simulink model "localization"  (R2019b)
settings: Solver=FixedStepAuto  StartTime=0.0  StopTime=310  FixedStep=sample_time  RelTol=1e-3
PreLoadFcn:
  | initLocalization
InitFcn:
  | initLocalization
  | insertArtificialOutages
StopFcn:
  | simout_data_prepared = false;
  | map_data_prepared = false;
  | % prepareSimOutData
undefined symbols (not defined in the file or in its folder): a_bias_gain, a_e_limit, a_e_ma_time, d_bogies, E_w_limit, E_w_ma_time, gnss_lever_arm, gnss_sample_time, gnss_speed_limit, imm_sample_time, p_llh_n_0_rad, psi_0, Q_arc, q_b_n_0, Q_imm, Q_imm_trash, Q_straight, sample_time, sigma_v_acc, sigma_v_gyro, v_min_tgc, v_ned_eb_n_0, w_bias_gain
libraries: libMdl_RecordedData x4, libMdl_quatToEuler x3, simulink x2, libMdl_InsBiasEstimator x2, libMdl_Imm x1, libMdl_KalmanFilter x1, libMdl_invQuat x1, libMdl_GnssDataCorrector x1, libMdl_ImuDataCorrector x1, libMdl_AccIntegrator x1, libMdl_AttitudeComputer x1, libMdl_CarriageMisalignment x1
(part 1 of 2)
settings Model: PauseTimes=14.4  Creator=Hanno  LastModifiedBy=wint_hn
settings SolverCC: AutoInsertRateTranBlk=on
settings DataIOCC: SaveOutput=off  SignalLogging=off  DSMLogging=off  SaveTime=off  ReturnWorkspaceOutputs=off

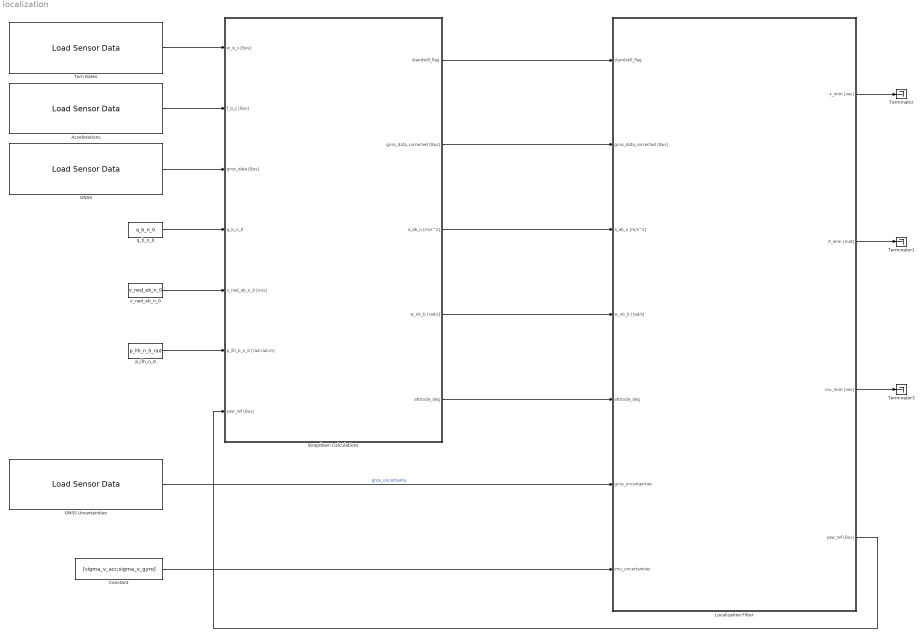
== system localization ==
  Accelerations : libMdl_RecordedData/Load Sensor Data  mv_input_data=acc_data  mv_data_validity=acc_data_validity  mv_input_time=time_imu  mv_sample_time=imu_sample_time
  Constant : Constant  Value=[sigma_v_acc;sigma_v_gyro]
  GNSS : libMdl_RecordedData/Load Sensor Data  mv_input_data=gnss_sim_data  mv_data_validity=gnss_sim_data_validity  mv_input_time=time_gnss  mv_sample_time=gnss_sample_time
  GNSS Uncertainties : libMdl_RecordedData/Load Sensor Data  mv_input_data=gnss_uncertainty_sim_data  mv_data_validity=gnss_sim_data_validity  mv_input_time=time_gnss  mv_sample_time=gnss_sample_time
  Localization Filter : Subsystem
  Strapdown Calculations : Subsystem
  Terminator : Terminator
  Terminator1 : Terminator
  Terminator3 : Terminator
  Turn Rates : libMdl_RecordedData/Load Sensor Data  mv_input_data=gyro_data  mv_data_validity=gyro_data_validity  mv_input_time=time_imu  mv_sample_time=imu_sample_time
  p_llh_n_0 : Constant  Value=p_llh_n_0_rad
  q_b_n_0 : Constant  Value=q_b_n_0
  v_ned_eb_n_0 : Constant  Value=v_ned_eb_n_0
  wires:
  Turn Rates/1 -> Strapdown Calculations/1(w_is_s [Bus])
  Accelerations/1 -> Strapdown Calculations/2(f_is_s [Bus])
  GNSS/1 -> Strapdown Calculations/3(gnss_data [Bus])
  q_b_n_0/1 -> Strapdown Calculations/4(q_b_n_0)
  v_ned_eb_n_0/1 -> Strapdown Calculations/5(v_ned_eb_n_0 [m/s])
  p_llh_n_0/1 -> Strapdown Calculations/6(p_llh_b_n_0 [rad,rad,m])
  Strapdown Calculations/2(gnss_data_corrected [Bus]) -> Localization Filter/2(gnss_data_corrected [Bus])
  GNSS Uncertainties/1 -> Localization Filter/6(gnss_uncertainties)  "gnss_uncertainty"
  Constant/1 -> Localization Filter/7(imu_uncertainties)
  Localization Filter/1(x_imm [vec]) -> Terminator/1
  Localization Filter/2(P_imm [mat]) -> Terminator1/1
  Localization Filter/3(mu_imm [vec]) -> Terminator3/1
  Strapdown Calculations/1(standstill_flag) -> Localization Filter/1(standstill_flag)
  Strapdown Calculations/3(a_eb_n [m/s^2]) -> Localization Filter/3(a_eb_n [m/s^2])
  Strapdown Calculations/4(w_nb_b [rad/s]) -> Localization Filter/4(w_nb_b [rad/s])
  Localization Filter/4(yaw_ref [Bus]) -> Strapdown Calculations/7(yaw_ref [Bus])
  Strapdown Calculations/5(attitude_deg) -> Localization Filter/5(attitude_deg)

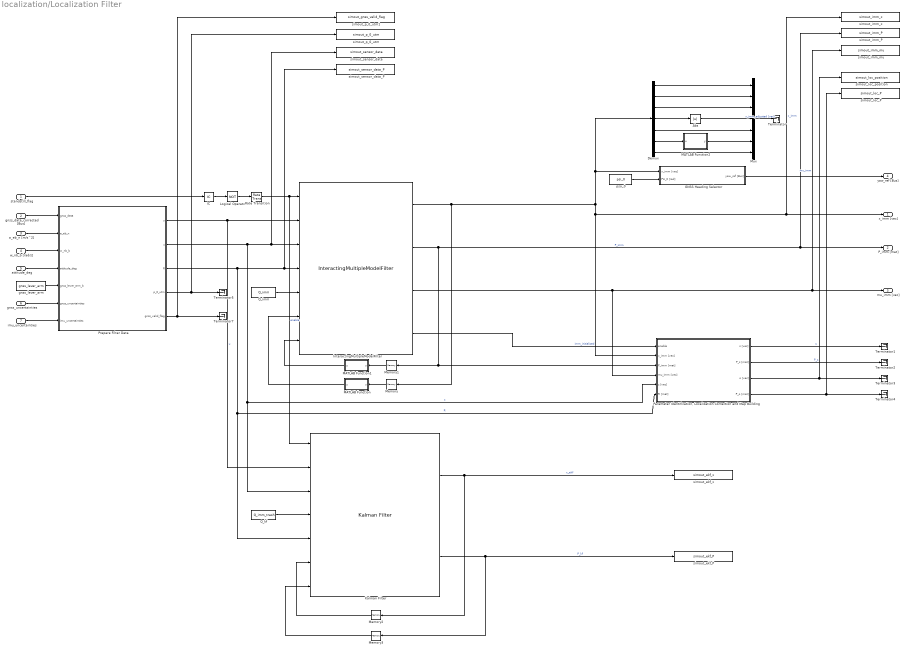
== system localization/Localization Filter ==
  standstill_flag : Inport
  gnss_data_corrected [Bus] : Inport  Port=2
  a_eb_n [m/s^2] : Inport  Port=3
  w_nb_b [rad/s] : Inport  Port=4
  attitude_deg : Inport  Port=5
  gnss_uncertainties : Inport  Port=6
  imu_uncertainties : Inport  Port=7
  Abs : Abs
  Demux : Demux  Outputs=7
  GNSS Heading Selector : Subsystem
  IC : InitialCondition
  InteractingMultipleModelFilter : libMdl_Imm/InteractingMultipleModelFilter  mv_sample_time=imm_sample_time  mv_mu_sample_time=imm_mu_sample_time  mv_x_0=x_0_imm  mv_P_0=P_0_imm  mv_pi=Pi  mv_mu_0=mu_0  mv_state_transition_functions=imm_state_transition_fcns  mv_measurement_functions=imm_measurement_fcns  mv_residuum_functions=imm_residuum_fcns
  Kalman Filter : libMdl_KalmanFilter/Kalman Filter  mv_sample_time=imm_sample_time  mv_x_0=x_0  mv_P_0=P_0  mv_state_transition_function=simFcn_Imm_Trash_StateTransitionFcn  mv_measurement_function=simFcn_Imm_MeasurementFcn  mv_residuum_function=simFcn_Imm_ResiduumFcn
  Logical Operator : Logic  Operator=NOT  AllPortsSameDT=off  OutDataTypeStr=boolean
  MATLAB Function : MATLAB Function  TreatAsAtomicUnit=on
  MATLAB Function1 : MATLAB Function  TreatAsAtomicUnit=on
  MATLAB Function2 : MATLAB Function  TreatAsAtomicUnit=on
  Memory{,1..3} (4 alike) : Memory
  Mux : Mux  Inputs=7
  "Parameter Identification, Localization Correction and Map Building" : Subsystem  TreatAsAtomicUnit=on  SystemSampleTime=imm_sample_time
  Prepare Filter Data : MATLAB Function  TreatAsAtomicUnit=on  SystemSampleTime=imm_sample_time
  Q_imm : Constant  Value=Q_imm
  Q_kf : Constant  Value=Q_imm_trash
  Rate Transition : RateTransition
  Terminator{,1..5,7} (7 alike) : Terminator
  gnss_lever_arm : Constant  Value=gnss_lever_arm
  pso_0 : Constant  Value=psi_0
  simout_ekf_P : ToWorkspace  VariableName=simout_ekf_P  SaveFormat=Timeseries  SampleTime=-1
  simout_ekf_x : ToWorkspace  VariableName=simout_ekf_x  SaveFormat=Timeseries  SampleTime=-1
  simout_imm_P : ToWorkspace  VariableName=simout_imm_P  SaveFormat=Timeseries  SampleTime=-1
  simout_imm_mu : ToWorkspace  VariableName=simout_imm_mu  SaveFormat=Timeseries  SampleTime=-1
  simout_imm_x : ToWorkspace  VariableName=simout_imm_x  SaveFormat=Timeseries  SampleTime=-1
  simout_loc_P : ToWorkspace  VariableName=simout_loc_P  SaveFormat=Timeseries  SampleTime=-1
  simout_loc_position : ToWorkspace  VariableName=simout_loc_position  SaveFormat=Timeseries  SampleTime=-1
  simout_p_0_utm : ToWorkspace  VariableName=simout_p_0_utm  SaveFormat=Timeseries  SampleTime=-1
      settings: MaxDataPoints=1
  simout_p_0_utm1 : ToWorkspace  VariableName=simout_gnss_valid_flag  SaveFormat=Timeseries  SampleTime=-1
  simout_sensor_data : ToWorkspace  VariableName=simout_sensor_data  SaveFormat=Timeseries  SampleTime=-1
  simout_sensor_data_P : ToWorkspace  VariableName=simout_sensor_data_P  SaveFormat=Timeseries  SampleTime=-1
  x_imm [vec] : Outport
  P_imm [mat] : Outport  Port=2
  mu_imm [vec] : Outport  Port=3
  yaw_ref [Bus] : Outport  Port=4
  wires:
  Q_imm/1 -> InteractingMultipleModelFilter/5
  Demux/1 -> Mux/1
  Demux/2 -> Mux/2
  Demux/3 -> Mux/3
  Demux/4 -> Abs/1
  Demux/5 -> Mux/5
  Demux/7 -> Mux/7
  Mux/1 -> Terminator/1  "x_imm_adjusted [vec]"
  Demux/6 -> MATLAB Function2/1(u)
  Abs/1 -> Mux/4
  Memory/1 -> MATLAB Function/1(u)
  MATLAB Function/1(y) -> InteractingMultipleModelFilter/6
  standstill_flag/1 -> IC/1
  MATLAB Function1/1(y) -> InteractingMultipleModelFilter/7
  Memory1/1 -> MATLAB Function1/1(u)
  Logical Operator/1 -> Rate Transition/1
  pso_0/1 -> GNSS Heading Selector/2(Psi_0 [rad])
  GNSS Heading Selector/1(yaw_ref [Bus]) -> yaw_ref [Bus]/1
  Prepare Filter Data/1(u) -> Kalman Filter/2, InteractingMultipleModelFilter/2  "u"
  Prepare Filter Data/2(z) -> Kalman Filter/3, "Parameter Identification, Localization Correction and Map Building"/5(z [vec]), simout_sensor_data/1, InteractingMultipleModelFilter/3  "z"
  Prepare Filter Data/3(R) -> Kalman Filter/5, "Parameter Identification, Localization Correction and Map Building"/6(R [mat]), simout_sensor_data_P/1, InteractingMultipleModelFilter/4  "R"
  gnss_data_corrected [Bus]/1 -> Prepare Filter Data/1(gnss_data)
  a_eb_n [m/s^2]/1 -> Prepare Filter Data/2(a_eb_n)
  w_nb_b [rad/s]/1 -> Prepare Filter Data/3(w_nb_b)
  gnss_uncertainties/1 -> Prepare Filter Data/6(gnss_uncertainties)
  imu_uncertainties/1 -> Prepare Filter Data/7(imu_uncertainties)
  InteractingMultipleModelFilter/3 -> simout_imm_mu/1, mu_imm [vec]/1, "Parameter Identification, Localization Correction and Map Building"/4(mu_imm [vec])  "mu_imm"
  InteractingMultipleModelFilter/2 -> simout_imm_P/1, P_imm [mat]/1, Memory1/1, "Parameter Identification, Localization Correction and Map Building"/3(P_imm [mat])  "P_imm"
  "Parameter Identification, Localization Correction and Map Building"/1(s [vec]) -> Terminator1/1  "s"
  InteractingMultipleModelFilter/1 -> Memory/1, Demux/1, GNSS Heading Selector/1(x_imm [vec]), simout_imm_x/1, x_imm [vec]/1, "Parameter Identification, Localization Correction and Map Building"/2(x_imm [vec])  "x_imm"
  "Parameter Identification, Localization Correction and Map Building"/2(P_s [mat]) -> Terminator2/1  "P_s"
  IC/1 -> Logical Operator/1
  Rate Transition/1 -> Kalman Filter/1, InteractingMultipleModelFilter/1  "enable"
  InteractingMultipleModelFilter/4 -> "Parameter Identification, Localization Correction and Map Building"/1(enable)  "imm_initialized"
  attitude_deg/1 -> Prepare Filter Data/4(attitude_deg)
  MATLAB Function2/1(y) -> Mux/6
  "Parameter Identification, Localization Correction and Map Building"/3(o [vec]) -> simout_loc_position/1, Terminator3/1
  "Parameter Identification, Localization Correction and Map Building"/4(P_o [mat]) -> simout_loc_P/1, Terminator4/1
  Prepare Filter Data/4(p_0_utm) -> simout_p_0_utm/1, Terminator5/1
  Prepare Filter Data/5(gnss_valid_flag) -> simout_p_0_utm1/1, Terminator7/1
  Memory2/1 -> Kalman Filter/6
  Kalman Filter/2 -> Memory3/1, simout_ekf_P/1  "P_kf"
  Memory3/1 -> Kalman Filter/7
  Q_kf/1 -> Kalman Filter/4
  Kalman Filter/1 -> simout_ekf_x/1, Memory2/1  "x_ekf"
  gnss_lever_arm/1 -> Prepare Filter Data/5(gnss_lever_arm_b)

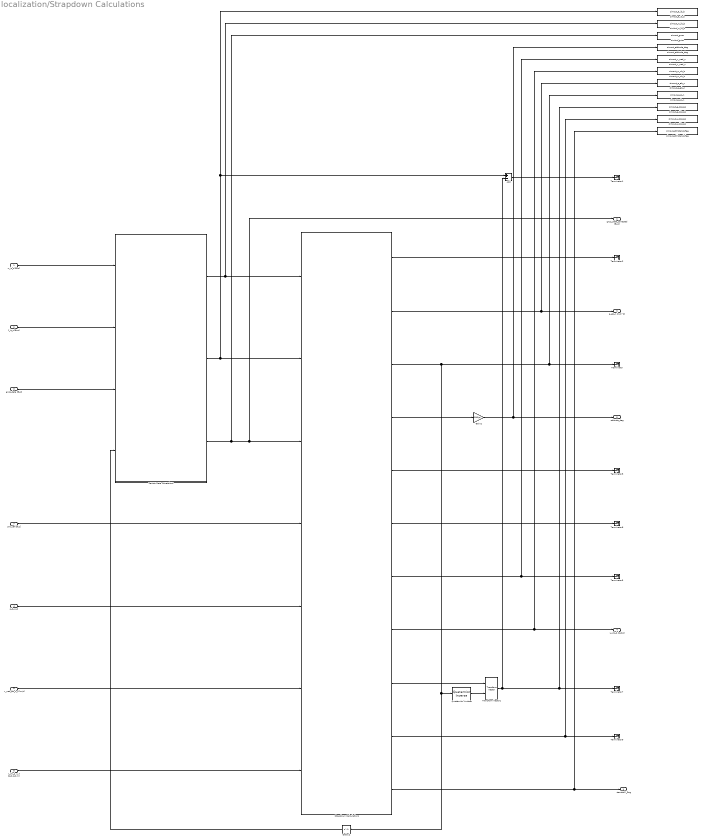
== system localization/Strapdown Calculations ==
  w_is_s [Bus] : Inport
  f_is_s [Bus] : Inport  Port=2
  gnss_data [Bus] : Inport  Port=3
  q_b_n_0 : Inport  Port=4
  v_ned_eb_n_0 [m/s] : Inport  Port=5
  p_llh_b_n_0 [rad,rad,m] : Inport  Port=6
  yaw_ref [Bus] : Inport  Port=7
  Add : Sum  Inputs=+-
  Delay2 : Delay  DelayLength=1  InitialCondition=q_b_n_0
  Gain2 : Gain  Gain=180/pi
      settings: AttributesFormatString=rad2deg
  Quaternion Inverse : libMdl_invQuat/Quaternion Inverse  SystemSampleTime=-1  Latency=0  AutoFrameSizeCalculation=off
  Sensor Data Corrections : Subsystem
  Strapdown Calculations : Subsystem
  Terminator{,1..3,5,7..9} (8 alike) : Terminator
  Transform Vector1 : libMdl_transformVect/Transform Vector  SystemSampleTime=-1  Latency=0  AutoFrameSizeCalculation=off
  simout_a_bias_b : ToWorkspace  VariableName=simout_a_bias_b  SaveFormat=Timeseries  SampleTime=-1
  simout_a_eb_n : ToWorkspace  VariableName=simout_a_eb_n  SaveFormat=Timeseries  SampleTime=-1
  simout_a_ib_b : ToWorkspace  VariableName=simout_a_ib_b  SaveFormat=Timeseries  SampleTime=-1
  simout_attitude_deg : ToWorkspace  VariableName=simout_attitude_deg  SaveFormat=Timeseries  SampleTime=-1
  simout_gnss : ToWorkspace  VariableName=simout_gnss  SaveFormat=Timeseries  SampleTime=-1
  simout_q_b_n : ToWorkspace  VariableName=simout_q_b_n  SaveFormat=Timeseries  SampleTime=-1
  simout_stillstand_flag : ToWorkspace  VariableName=simout_stillstand_flag  SaveFormat=Timeseries  SampleTime=-1
  simout_v_ned_n : ToWorkspace  VariableName=simout_v_ned_n  SaveFormat=Timeseries  SampleTime=-1
  simout_w_bias_b : ToWorkspace  VariableName=simout_w_bias_b  SaveFormat=Timeseries  SampleTime=-1
  simout_w_ib_b : ToWorkspace  VariableName=simout_w_ib_b  SaveFormat=Timeseries  SampleTime=-1
  simout_w_nb_b : ToWorkspace  VariableName=simout_w_nb_b  SaveFormat=Timeseries  SampleTime=-1
  standstill_flag : Outport
  gnss_data_corrected [Bus] : Outport  Port=2
  a_eb_n [m/s^2] : Outport  Port=3
  w_nb_b [rad/s] : Outport  Port=4
  attitude_deg : Outport  Port=5
  wires:
  Strapdown Calculations/10(w_bias_b [rad/s]) -> simout_w_bias_b/1, Terminator9/1  "w_bias_b"
  Strapdown Calculations/6(w_nb_b_raw [rad/s]) -> Terminator8/1  "w_nb_b_raw"
  p_llh_b_n_0 [rad,rad,m]/1 -> Strapdown Calculations/7(p_llh_b_n_0 [rad,rad,m])
  Sensor Data Corrections/3(gnss_data_corrected [Bus]) -> simout_gnss/1, gnss_data_corrected [Bus]/1, Strapdown Calculations/3(gnss_data [Bus])  "gnss_data_corrected"
  Strapdown Calculations/3(q_b_n) -> simout_q_b_n/1, Terminator/1, Delay2/1, Quaternion Inverse/1  "q_b_n"
  Gain2/1 -> attitude_deg/1, simout_attitude_deg/1  "attitude_deg"
  Strapdown Calculations/4(E_b_n [rad]) -> Gain2/1
  Strapdown Calculations/8(w_nb_b [rad/s]) -> simout_w_nb_b/1, w_nb_b [rad/s]/1  "w_nb_b"
  Strapdown Calculations/7(v_ned_eb_n [m/s]) -> Terminator5/1, simout_v_ned_n/1  "v_ned_eb_n"
  Strapdown Calculations/2(a_eb_n [m/s^2]) -> simout_a_eb_n/1, a_eb_n [m/s^2]/1  "a_eb_n"
  Quaternion Inverse/1 -> Transform Vector1/2
  Sensor Data Corrections/1(w_ib_b [rad/s]) -> simout_w_ib_b/1, Strapdown Calculations/1(w_ib_b [rad/s])  "w_ib_b"
  v_ned_eb_n_0 [m/s]/1 -> Strapdown Calculations/6(v_ned_eb_n_0 [m/s])
  Strapdown Calculations/1("p_llh_b_n [deg, deg, m]") -> Terminator2/1  "p_llh_b_n [deg,deg,m]"
  Strapdown Calculations/5(a_eb_n_raw [m/s^2]) -> Terminator3/1  "a_eb_n_raw"
  Strapdown Calculations/11(standstill_flag) -> simout_stillstand_flag/1, standstill_flag/1  "standstill_flag"
  Transform Vector1/1 -> Terminator7/1, simout_a_bias_b/1, Add/2  "a_bias_b"
  Strapdown Calculations/9(a_bias_n [m/s^2]) -> Transform Vector1/1
  q_b_n_0/1 -> Strapdown Calculations/5(q_b_n_0)
  w_is_s [Bus]/1 -> Sensor Data Corrections/1(w_is_s [Bus])
  f_is_s [Bus]/1 -> Sensor Data Corrections/2(f_is_s [Bus])
  gnss_data [Bus]/1 -> Sensor Data Corrections/3(gnss_data [Bus])
  Delay2/1 -> Sensor Data Corrections/4(q_b_n)
  Sensor Data Corrections/2(f_ib_b [m/s^2]) -> Add/1, simout_a_ib_b/1, Strapdown Calculations/2(f_ib_b [m/s^2])
  Add/1 -> Terminator1/1  "f_ib_b_corrected"
  yaw_ref [Bus]/1 -> Strapdown Calculations/4(yaw_ref [Bus])

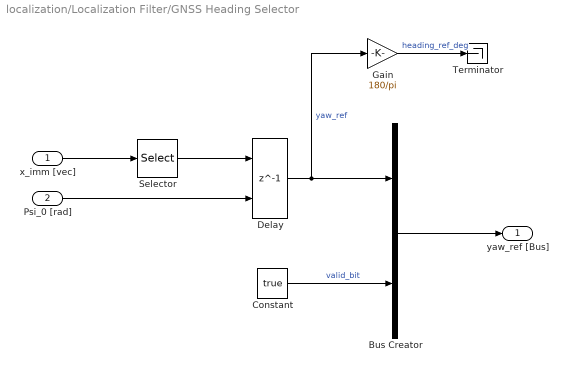
== system localization/Localization Filter/GNSS Heading Selector ==
  x_imm [vec] : Inport
  Psi_0 [rad] : Inport  Port=2
  Bus Creator : BusCreator  Inputs=2
  Constant : Constant  Value=true
  Delay : Delay  DelayLength=1  InitialConditionSource=Input port  InitialCondition=0
      settings: InputPortMap=u0,p4
  Gain : Gain  Gain=180/pi
  Selector : Selector  InputPortWidth=7  IndexOptions=Index vector (dialog)  Indices=6  OutputSizes=1
  Terminator : Terminator
  yaw_ref [Bus] : Outport
  wires:
  Bus Creator/1 -> yaw_ref [Bus]/1
  Selector/1 -> Delay/1
  x_imm [vec]/1 -> Selector/1
  Constant/1 -> Bus Creator/2  "valid_bit"
  Delay/1 -> Gain/1, Bus Creator/1  "yaw_ref"
  Psi_0 [rad]/1 -> Delay/2
  Gain/1 -> Terminator/1  "heading_ref_deg"

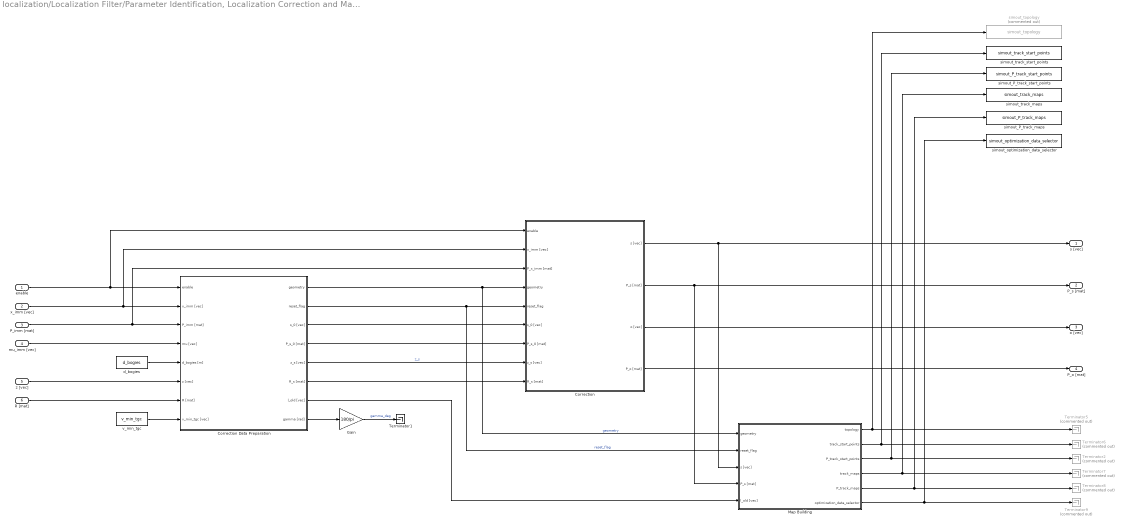
== system localization/Localization Filter/Parameter Identification, Localization Correction and Map Building ==
  enable : Inport
  x_imm [vec] : Inport  Port=2
  P_imm [mat] : Inport  Port=3
  mu_imm [vec] : Inport  Port=4
  z [vec] : Inport  Port=5
  R [mat] : Inport  Port=6
  Correction : Subsystem
  Correction Data Preparation : Subsystem
  Gain : Gain  Gain=180/pi
  Map Building : Subsystem
  Terminator1 : Terminator
  Terminator{2,5..9} (6 alike) : Terminator  Commented=on
  d_bogies : Constant  Value=d_bogies
  simout_P_track_maps : ToWorkspace  VariableName=simout_P_track_maps  SaveFormat=Structure With Time  SampleTime=-1
      settings: MaxDataPoints=1
  simout_P_track_start_points : ToWorkspace  VariableName=simout_P_track_start_points  SaveFormat=Structure With Time  SampleTime=-1
      settings: MaxDataPoints=1
  simout_optimization_data_selector : ToWorkspace  VariableName=simout_optimization_data_selector  SaveFormat=Structure With Time  SampleTime=-1
      settings: MaxDataPoints=1
  simout_topology : ToWorkspace  Commented=on  VariableName=simout_topology  SaveFormat=Structure With Time  SampleTime=-1
      settings: MaxDataPoints=1
  simout_track_maps : ToWorkspace  VariableName=simout_track_maps  SaveFormat=Structure With Time  SampleTime=-1
      settings: MaxDataPoints=1
  simout_track_start_points : ToWorkspace  VariableName=simout_track_start_points  SaveFormat=Structure With Time  SampleTime=-1
      settings: MaxDataPoints=1
  v_min_tgc : Constant  Value=v_min_tgc
  s [vec] : Outport  VectorParamsAs1DForOutWhenUnconnected=off
  P_s [mat] : Outport  Port=2  VectorParamsAs1DForOutWhenUnconnected=off
  o [vec] : Outport  Port=3  VectorParamsAs1DForOutWhenUnconnected=off
  P_o [mat] : Outport  Port=4  VectorParamsAs1DForOutWhenUnconnected=off
  wires:
  Correction Data Preparation/2(reset_flag) -> Map Building/2(reset_flag), Correction/5(reset_flag)  "reset_flag"
  P_imm [mat]/1 -> Correction/3(P_x_imm [mat]), Correction Data Preparation/3(P_imm [mat])
  Correction Data Preparation/6(R_s [mat]) -> Correction/9(R_s [mat])
  Correction Data Preparation/3(s_0 [vec]) -> Correction/6(s_0 [vec])
  Correction Data Preparation/4(P_s_0 [mat]) -> Correction/7(P_s_0 [mat])
  Correction/2(P_s [mat]) -> Map Building/4(P_s [mat]), P_s [mat]/1
  mu_imm [vec]/1 -> Correction Data Preparation/4(mu [vec])
  Correction/1(s [vec]) -> Map Building/3(s [vec]), s [vec]/1
  Correction Data Preparation/5(z_s [vec]) -> Correction/8(z_s [vec])  "z_s"
  x_imm [vec]/1 -> Correction/2(x_imm [vec]), Correction Data Preparation/2(x_imm [vec])
  Correction Data Preparation/1(geometry) -> Map Building/1(geometry), Correction/4(geometry)  "geometry"
  enable/1 -> Correction/1(enable), Correction Data Preparation/1(enable)
  Gain/1 -> Terminator1/1  "gamma_deg"
  Correction Data Preparation/8(gamma [rad]) -> Gain/1
  d_bogies/1 -> Correction Data Preparation/5(d_bogies [m])
  Correction/3(o [vec]) -> o [vec]/1
  Correction/4(P_o [mat]) -> P_o [mat]/1
  Map Building/5(P_track_maps) -> simout_P_track_maps/1, Terminator8/1
  Map Building/2(track_start_points) -> simout_track_start_points/1, Terminator6/1
  Map Building/1(topology) -> simout_topology/1, Terminator5/1
  Map Building/4(track_maps) -> simout_track_maps/1, Terminator7/1
  Map Building/6(optimization_data_selector) -> simout_optimization_data_selector/1, Terminator9/1
  Map Building/3(P_track_start_points) -> simout_P_track_start_points/1, Terminator2/1
  z [vec]/1 -> Correction Data Preparation/6(z [vec])
  R [mat]/1 -> Correction Data Preparation/7(R [mat])
  v_min_tgc/1 -> Correction Data Preparation/8(v_min_tgc [vec])
  Correction Data Preparation/7(l_old [vec]) -> Map Building/5(l_old [vec])

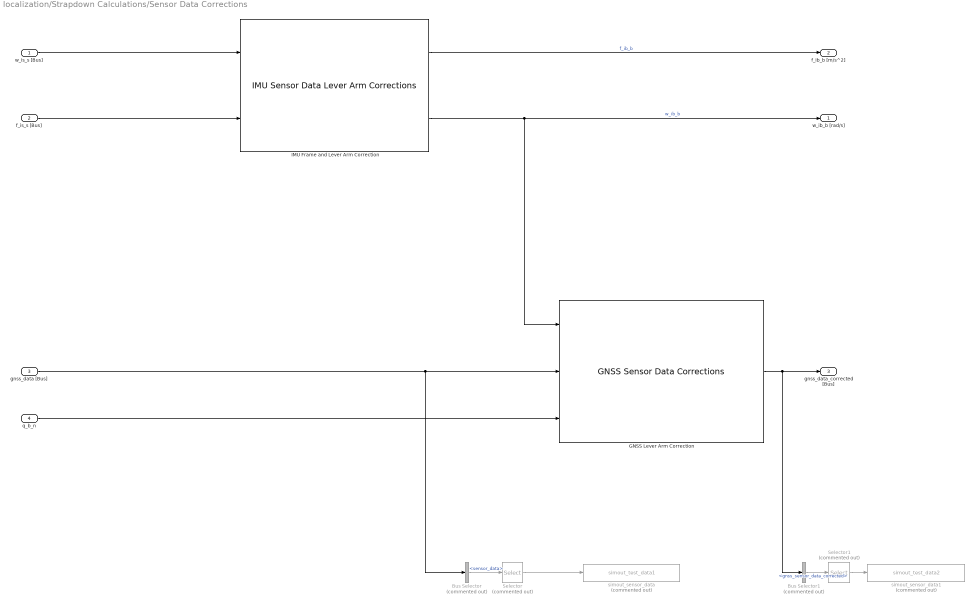
== system localization/Strapdown Calculations/Sensor Data Corrections ==
  w_is_s [Bus] : Inport
  f_is_s [Bus] : Inport  Port=2
  gnss_data [Bus] : Inport  Port=3
  q_b_n : Inport  Port=4
  Bus Selector : BusSelector  Commented=on  OutputSignals=sensor_data
  Bus Selector1 : BusSelector  Commented=on  OutputSignals=gnss_sensor_data_corrected
  GNSS Lever Arm Correction : libMdl_GnssDataCorrector/GNSS Sensor Data Corrections  mv_lever_arm=gnss_lever_arm  mv_sample_time=sample_time  mv_position_correction=on
  IMU Frame and Lever Arm Correction : libMdl_ImuDataCorrector/IMU Sensor Data Lever Arm Corrections  mv_lever_arm=imu_lever_arm  mv_mounting_attitude=[1;0;0;0]  mv_enable_euler_correction=off  mv_euler_ma_time=f_euler_ma_time  mv_sample_time=sample_time
  Selector : Selector  Commented=on  InputPortWidth=7  IndexOptions=Index vector (dialog)  Indices=1:2  OutputSizes=1
  Selector1 : Selector  Commented=on  InputPortWidth=7  IndexOptions=Index vector (dialog)  Indices=1:2  OutputSizes=1
  simout_sensor_data : ToWorkspace  Commented=on  VariableName=simout_test_data1  SaveFormat=Timeseries  SampleTime=-1
  simout_sensor_data1 : ToWorkspace  Commented=on  VariableName=simout_test_data2  SaveFormat=Timeseries  SampleTime=-1
  w_ib_b [rad/s] : Outport
  f_ib_b [m/s^2] : Outport  Port=2
  gnss_data_corrected [Bus] : Outport  Port=3
  wires:
  IMU Frame and Lever Arm Correction/2 -> w_ib_b [rad/s]/1, GNSS Lever Arm Correction/1  "w_ib_b"
  q_b_n/1 -> GNSS Lever Arm Correction/3
  gnss_data [Bus]/1 -> Bus Selector/1, GNSS Lever Arm Correction/2
  IMU Frame and Lever Arm Correction/1 -> f_ib_b [m/s^2]/1  "f_ib_b"
  w_is_s [Bus]/1 -> IMU Frame and Lever Arm Correction/1
  f_is_s [Bus]/1 -> IMU Frame and Lever Arm Correction/2
  Bus Selector/1 -> Selector/1  "<sensor_data>"
  Selector/1 -> simout_sensor_data/1
  GNSS Lever Arm Correction/1 -> Bus Selector1/1, gnss_data_corrected [Bus]/1
  Bus Selector1/1 -> Selector1/1  "<gnss_sensor_data_corrected>"
  Selector1/1 -> simout_sensor_data1/1

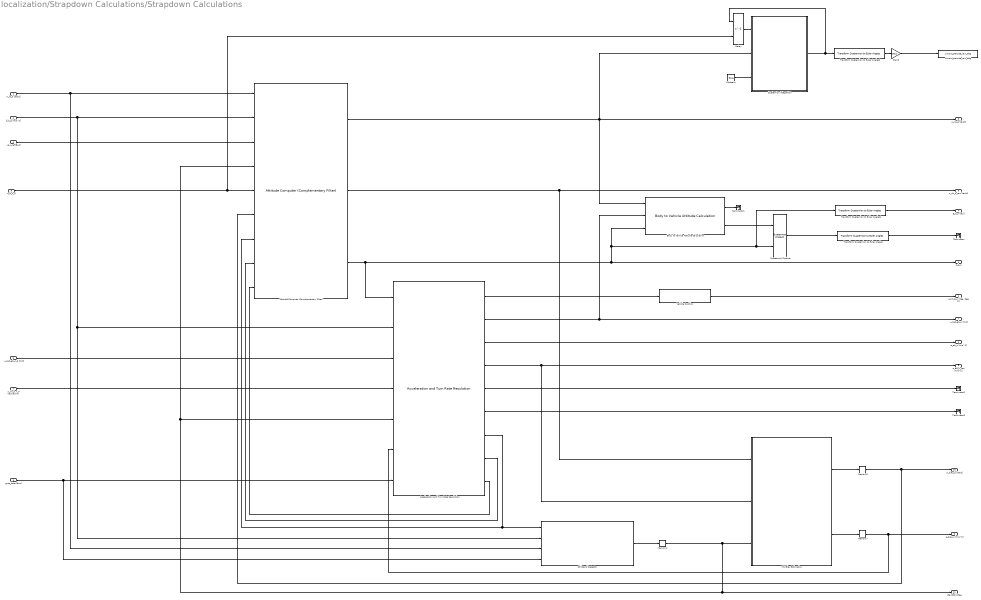
== system localization/Strapdown Calculations/Strapdown Calculations ==
  w_ib_b [rad/s] : Inport
  f_ib_b [m/s^2] : Inport  Port=2
  gnss_data [Bus] : Inport  Port=3
  yaw_ref [Bus] : Inport  Port=4
  q_b_n_0 : Inport  Port=5
  v_ned_eb_n_0 [m/s] : Inport  Port=6
  p_llh_b_n_0 [rad,rad,m] : Inport  Port=7
  "Acceleration and Turn Rate Resulotion " : libMdl_AccIntegrator/Acceleration and Turn Rate Resulotion   mv_sample_time=-1
  Attitude Computer (Complementary Filter) : libMdl_AttitudeComputer/Attitude Computer (Complementary Filter)  mv_static_alpha=comp_filter_static_gain  mv_adaptive_gain_thresholds=comp_filter_adaptive_gain_thresholds  mv_enable_heading_correction=on  mv_sample_time=-1
      settings: AttributesFormatString="see: Valenti et al., \"Keeping a Good Attitude: A Quaternion-Based Orientation Filter for IMUs and MARGs\", Sensors, pp. 19302-19330, 2015"
  Body to Vehicle Attitude Calculation : libMdl_CarriageMisalignment/Body to Vehicle Attitude Calculation  mv_d_bogies=15.1
  Constant : Constant  Value=false
  Delay : Delay  DelayLength=1  InitialConditionSource=Input port
      settings: InputPortMap=u0,p4
  Gain3 : Gain  Gain=180/pi
      settings: AttributesFormatString=rad2deg
  IMU Bias Estimation : Subsystem  mask(IMU Bias Estimation){mv_gyro_bias_gain=w_bias_gain, mv_acc_bias_gain=a_bias_gain}
      mask prompts: mv_gyro_bias_gain "Gyro Bias Gain:"; mv_acc_bias_gain "Acc. Bias Gain:"
      mask Display:
      | str1 = sprintf('\\color{black}{\\bfIMU Bias Estimation}\n\n');
      | str2 = sprintf('Gyro Bias Gain: %0.6f\n',mv_gyro_bias_gain);
      | str3 = sprintf('Acc. Bias Gain: %0.6f',mv_acc_bias_gain);
      | 
      | str = [str1,str2,str3];
      | 
      | text( 0.5,0.5, ...
      |       str, ...
      |       'horizontalAlignment', 'center', ...
      |       'texmode','on' ...
      |     )
  Memory1 : Memory
  Memory7 : Memory
  Memory8 : Memory
  Quaternion Integration : Subsystem
      settings: AttributesFormatString="See:  D. Titterton and J. Westen, \"Strapdown Inertial Navigation Technology\", pp. 319-320, IET, 2004"
  Quaternion Product : libMdl_multQuat/Quaternion Product  SystemSampleTime=-1  Latency=0  AutoFrameSizeCalculation=off
  Stillstand Detector : Subsystem  mask(Standstill Detection){mv_w_energy_standstill_limit=E_w_limit, mv_E_w_ma_time=E_w_ma_time, mv_acc_limit=a_e_limit, mv_a_e_ma_time=a_e_ma_time, mv_gnss_speed_limit=gnss_speed_limit}
      mask prompts: mv_w_energy_standstill_limit "Turn Rate Standstill Energy Limit:"; mv_E_w_ma_time "Turn Rate Energy Averaging Time:"; mv_acc_limit "Acceleration Limit:"; mv_a_e_ma_time "Acceleration Averaging Time:"; mv_gnss_speed_limit "GNSS Speed Limit:"
      mask Display:
      | str1 = sprintf('\\color{black}{\\bfStillstand Detector}\n\n');
      | str2 = sprintf('Turn Rate Energy Limit: %.1e\n',mv_w_energy_standstill_limit);
      | str3 = sprintf('Turn Rate Energy Averaging Time: %.1f\n',mv_E_w_ma_time);
      | str4 = sprintf('Acceleration Limit: %.1e\n',mv_acc_limit);
      | str5 = sprintf('Acceleration Averaging Time: %.1f\n',mv_a_e_ma_time);
      | str6 = sprintf('GNSS Speed Limit: %.1f',mv_gnss_speed_limit);
      | 
      | str = [str1,str2,str3,str4,str5,str6];
      | 
      | text( 0.5,0.5, ...
      |       str, ...
      |       'horizontalAlignment', 'center', ...
      |       'texmode','on' ...
      |     )
  Terminator{,1..3} (4 alike) : Terminator
  Transform Quaternion to Euler Angles : libMdl_quatToEuler/Transform Quaternion to Euler Angles  SystemSampleTime=-1  Latency=0  AutoFrameSizeCalculation=off
  Transform Quaternion to Euler Angles1 : libMdl_quatToEuler/Transform Quaternion to Euler Angles  SystemSampleTime=-1  Latency=0  AutoFrameSizeCalculation=off
  Transform Quaternion to Euler Angles2 : libMdl_quatToEuler/Transform Quaternion to Euler Angles  SystemSampleTime=-1  Latency=0  AutoFrameSizeCalculation=off
  Vehicle Position : Subsystem
  simout_attitude_raw_deg : ToWorkspace  VariableName=simout_attitude_raw_deg  SaveFormat=Timeseries  SampleTime=-1
  "p_llh_b_n [deg, deg, m]" : Outport
  a_eb_n [m/s^2] : Outport  Port=2
  q_b_n : Outport  Port=3
  E_b_n [rad] : Outport  Port=4
  a_eb_n_raw [m/s^2] : Outport  Port=5
  w_nb_b_raw [rad/s] : Outport  Port=6
  v_ned_eb_n [m/s] : Outport  Port=7
  w_nb_b [rad/s] : Outport  Port=8
  a_bias_n [m/s^2] : Outport  Port=9
  w_bias_b [rad/s] : Outport  Port=10
  standstill_flag : Outport  Port=11
  wires:
  Vehicle Position/1("p_llh_b_n [deg, deg, m]") -> "p_llh_b_n [deg, deg, m]"/1
  "Acceleration and Turn Rate Resulotion "/2 -> v_ned_eb_n [m/s]/1, Body to Vehicle Attitude Calculation/2
  "Acceleration and Turn Rate Resulotion "/1 -> Vehicle Position/1("p_llh_b_n [rad, rad, m]")
  "Acceleration and Turn Rate Resulotion "/5 -> Terminator2/1
  "Acceleration and Turn Rate Resulotion "/6 -> Terminator3/1
  Attitude Computer (Complementary Filter)/2 -> w_nb_b_raw [rad/s]/1, IMU Bias Estimation/1(w_nb_b_raw [rad/s])  "w_nb_b_raw"
  "Acceleration and Turn Rate Resulotion "/4 -> IMU Bias Estimation/2(a_eb_n_raw [m/s^2]), a_eb_n_raw [m/s^2]/1
  p_llh_b_n_0 [rad,rad,m]/1 -> "Acceleration and Turn Rate Resulotion "/4
  v_ned_eb_n_0 [m/s]/1 -> "Acceleration and Turn Rate Resulotion "/3
  "Acceleration and Turn Rate Resulotion "/9 -> Attitude Computer (Complementary Filter)/9
  "Acceleration and Turn Rate Resulotion "/8 -> Attitude Computer (Complementary Filter)/8
  "Acceleration and Turn Rate Resulotion "/7 -> Attitude Computer (Complementary Filter)/7, Stillstand Detector/1(f_local_gravity [m/s^2])
  IMU Bias Estimation/1(w_nb_b_bias [rad/s]) -> Memory8/1  "w_nb_b_bias"
  IMU Bias Estimation/2(a_eb_n_bias [m/s^2]) -> Memory7/1  "a_eb_n_bias"
  Body to Vehicle Attitude Calculation/2 -> Quaternion Product/1
  Quaternion Product/1 -> Transform Quaternion to Euler Angles/1
  Body to Vehicle Attitude Calculation/1 -> Terminator1/1  "alpha"
  Attitude Computer (Complementary Filter)/3 -> "Acceleration and Turn Rate Resulotion "/1, q_b_n/1, Body to Vehicle Attitude Calculation/3, Transform Quaternion to Euler Angles1/1, Quaternion Product/2
  Transform Quaternion to Euler Angles1/1 -> E_b_n [rad]/1
  Transform Quaternion to Euler Angles/1 -> Terminator/1
  "Acceleration and Turn Rate Resulotion "/3 -> a_eb_n [m/s^2]/1
  Memory8/1 -> w_bias_b [rad/s]/1, Attitude Computer (Complementary Filter)/6
  Memory7/1 -> "Acceleration and Turn Rate Resulotion "/6, a_bias_n [m/s^2]/1
  Stillstand Detector/1(standstill_flag) -> Memory1/1  "standstill_flag"
  gnss_data [Bus]/1 -> "Acceleration and Turn Rate Resulotion "/7, Stillstand Detector/4(gnss_data [Bus])
  yaw_ref [Bus]/1 -> Attitude Computer (Complementary Filter)/3
  q_b_n_0/1 -> Attitude Computer (Complementary Filter)/5, Delay/2
  Memory1/1 -> IMU Bias Estimation/3(stillstand_flag), "Acceleration and Turn Rate Resulotion "/5, Attitude Computer (Complementary Filter)/4, standstill_flag/1
  Quaternion Integration/1(q_b_n) -> Delay/1, Transform Quaternion to Euler Angles2/1
  Constant/1 -> Quaternion Integration/3(standstill_flag)
  Gain3/1 -> simout_attitude_raw_deg/1
  w_ib_b [rad/s]/1 -> Stillstand Detector/3(w_ib_b [rad/s]), Attitude Computer (Complementary Filter)/1
  Transform Quaternion to Euler Angles2/1 -> Gain3/1
  Attitude Computer (Complementary Filter)/1 -> Quaternion Integration/2(w_nb_b [rad/s]), Body to Vehicle Attitude Calculation/1, w_nb_b [rad/s]/1
  Delay/1 -> Quaternion Integration/1(q_b_n_prev)
  f_ib_b [m/s^2]/1 -> Attitude Computer (Complementary Filter)/2, "Acceleration and Turn Rate Resulotion "/2, Stillstand Detector/2(f_ib_b [m/s^2])

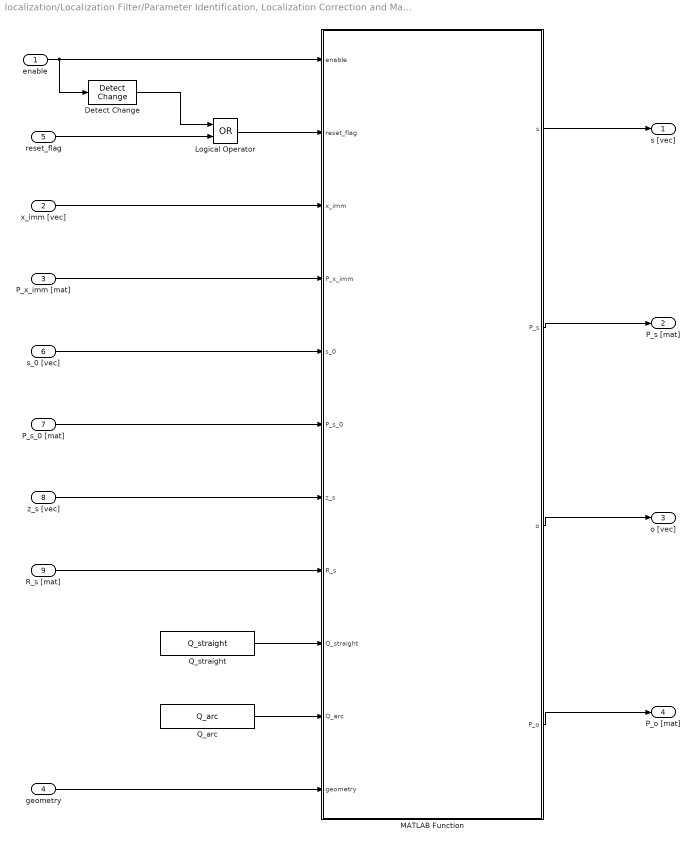
== system localization/Localization Filter/Parameter Identification, Localization Correction and Map Building/Correction ==
  enable : Inport
  x_imm [vec] : Inport  Port=2
  P_x_imm [mat] : Inport  Port=3
  geometry : Inport  Port=4
  reset_flag : Inport  Port=5
  s_0 [vec] : Inport  Port=6
  P_s_0 [mat] : Inport  Port=7
  z_s [vec] : Inport  Port=8
  R_s [mat] : Inport  Port=9
  Detect Change : simulink/Logic and Bit Operations/Detect Change  vinit=0  OutDataTypeStr=boolean
  Logical Operator : Logic  Operator=OR  AllPortsSameDT=off  OutDataTypeStr=boolean
  MATLAB Function : MATLAB Function  TreatAsAtomicUnit=on
  Q_arc : Constant  Value=Q_arc
  Q_straight : Constant  Value=Q_straight
  s [vec] : Outport  VectorParamsAs1DForOutWhenUnconnected=off
  P_s [mat] : Outport  Port=2  VectorParamsAs1DForOutWhenUnconnected=off
  o [vec] : Outport  Port=3  VectorParamsAs1DForOutWhenUnconnected=off
  P_o [mat] : Outport  Port=4  VectorParamsAs1DForOutWhenUnconnected=off
  wires:
  geometry/1 -> MATLAB Function/11(geometry)
  MATLAB Function/1(s) -> s [vec]/1
  MATLAB Function/2(P_s) -> P_s [mat]/1
  s_0 [vec]/1 -> MATLAB Function/5(s_0)
  P_s_0 [mat]/1 -> MATLAB Function/6(P_s_0)
  reset_flag/1 -> Logical Operator/2
  x_imm [vec]/1 -> MATLAB Function/3(x_imm)
  P_x_imm [mat]/1 -> MATLAB Function/4(P_x_imm)
  z_s [vec]/1 -> MATLAB Function/7(z_s)
  R_s [mat]/1 -> MATLAB Function/8(R_s)
  enable/1 -> Detect Change/1, MATLAB Function/1(enable)
  Detect Change/1 -> Logical Operator/1
  Logical Operator/1 -> MATLAB Function/2(reset_flag)
  MATLAB Function/3(o) -> o [vec]/1
  MATLAB Function/4(P_o) -> P_o [mat]/1
  Q_straight/1 -> MATLAB Function/9(Q_straight)
  Q_arc/1 -> MATLAB Function/10(Q_arc)

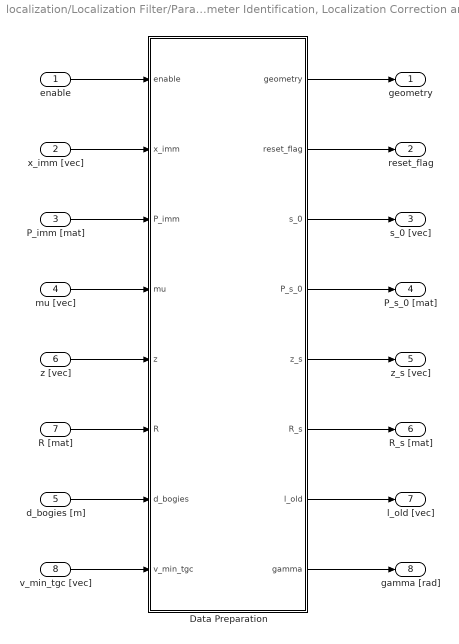
== system localization/Localization Filter/Parameter Identification, Localization Correction and Map Building/Correction Data Preparation ==
  enable : Inport
  x_imm [vec] : Inport  Port=2
  P_imm [mat] : Inport  Port=3
  mu [vec] : Inport  Port=4
  d_bogies [m] : Inport  Port=5
  z [vec] : Inport  Port=6
  R [mat] : Inport  Port=7
  v_min_tgc [vec] : Inport  Port=8
  Data Preparation : MATLAB Function  TreatAsAtomicUnit=on
  geometry : Outport  VectorParamsAs1DForOutWhenUnconnected=off
  reset_flag : Outport  Port=2  VectorParamsAs1DForOutWhenUnconnected=off
  s_0 [vec] : Outport  Port=3  VectorParamsAs1DForOutWhenUnconnected=off
  P_s_0 [mat] : Outport  Port=4  VectorParamsAs1DForOutWhenUnconnected=off
  z_s [vec] : Outport  Port=5  VectorParamsAs1DForOutWhenUnconnected=off
  R_s [mat] : Outport  Port=6  VectorParamsAs1DForOutWhenUnconnected=off
  l_old [vec] : Outport  Port=7  VectorParamsAs1DForOutWhenUnconnected=off
  gamma [rad] : Outport  Port=8  VectorParamsAs1DForOutWhenUnconnected=off
  wires:
  P_imm [mat]/1 -> Data Preparation/3(P_imm)
  mu [vec]/1 -> Data Preparation/4(mu)
  x_imm [vec]/1 -> Data Preparation/2(x_imm)
  Data Preparation/1(geometry) -> geometry/1
  Data Preparation/2(reset_flag) -> reset_flag/1
  Data Preparation/3(s_0) -> s_0 [vec]/1
  Data Preparation/4(P_s_0) -> P_s_0 [mat]/1
  Data Preparation/5(z_s) -> z_s [vec]/1
  Data Preparation/6(R_s) -> R_s [mat]/1
  d_bogies [m]/1 -> Data Preparation/7(d_bogies)
  Data Preparation/8(gamma) -> gamma [rad]/1
  enable/1 -> Data Preparation/1(enable)
  R [mat]/1 -> Data Preparation/6(R)
  z [vec]/1 -> Data Preparation/5(z)
  v_min_tgc [vec]/1 -> Data Preparation/8(v_min_tgc)
  Data Preparation/7(l_old) -> l_old [vec]/1

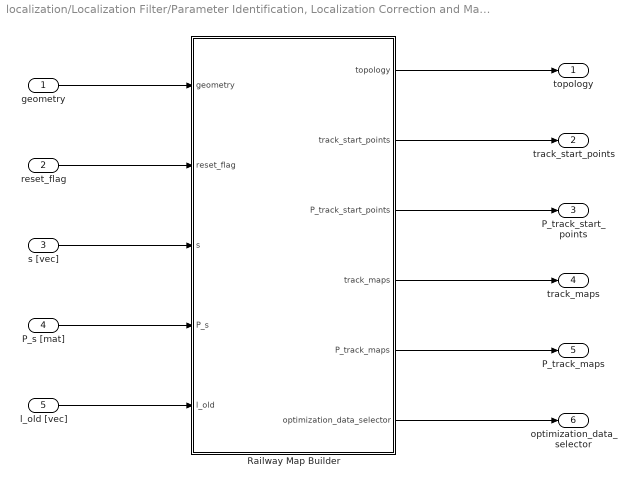
== system localization/Localization Filter/Parameter Identification, Localization Correction and Map Building/Map Building ==
  geometry : Inport
  reset_flag : Inport  Port=2
  s [vec] : Inport  Port=3
  P_s [mat] : Inport  Port=4
  l_old [vec] : Inport  Port=5
  Railway Map Builder : MATLAB Function  TreatAsAtomicUnit=on
  topology : Outport  VectorParamsAs1DForOutWhenUnconnected=off
  track_start_points : Outport  Port=2  VectorParamsAs1DForOutWhenUnconnected=off
  P_track_start_points : Outport  Port=3  VectorParamsAs1DForOutWhenUnconnected=off
  track_maps : Outport  Port=4  VectorParamsAs1DForOutWhenUnconnected=off
  P_track_maps : Outport  Port=5  VectorParamsAs1DForOutWhenUnconnected=off
  optimization_data_selector : Outport  Port=6  VectorParamsAs1DForOutWhenUnconnected=off
  wires:
  geometry/1 -> Railway Map Builder/1(geometry)
  reset_flag/1 -> Railway Map Builder/2(reset_flag)
  s [vec]/1 -> Railway Map Builder/3(s)
  P_s [mat]/1 -> Railway Map Builder/4(P_s)
  Railway Map Builder/6(optimization_data_selector) -> optimization_data_selector/1
  Railway Map Builder/5(P_track_maps) -> P_track_maps/1
  Railway Map Builder/1(topology) -> topology/1
  Railway Map Builder/2(track_start_points) -> track_start_points/1
  Railway Map Builder/4(track_maps) -> track_maps/1
  Railway Map Builder/3(P_track_start_points) -> P_track_start_points/1
  l_old [vec]/1 -> Railway Map Builder/5(l_old)

== system localization/Strapdown Calculations/Strapdown Calculations/IMU Bias Estimation ==
  w_nb_b_raw [rad/s] : Inport
  a_eb_n_raw [m/s^2] : Inport  Port=2
  stillstand_flag : Inport  Port=3
  Acceleration Bias Estimator : libMdl_InsBiasEstimator/Bias Estimator  mv_bias_gain=mv_acc_bias_gain
  Turn Rate Bias Estimator : libMdl_InsBiasEstimator/Bias Estimator  mv_bias_gain=mv_gyro_bias_gain
  w_nb_b_bias [rad/s] : Outport
  a_eb_n_bias [m/s^2] : Outport  Port=2
  wires:
  a_eb_n_raw [m/s^2]/1 -> Acceleration Bias Estimator/1
  Turn Rate Bias Estimator/1 -> w_nb_b_bias [rad/s]/1
  stillstand_flag/1 -> Acceleration Bias Estimator/2, Turn Rate Bias Estimator/2
  w_nb_b_raw [rad/s]/1 -> Turn Rate Bias Estimator/1
  Acceleration Bias Estimator/1 -> a_eb_n_bias [m/s^2]/1

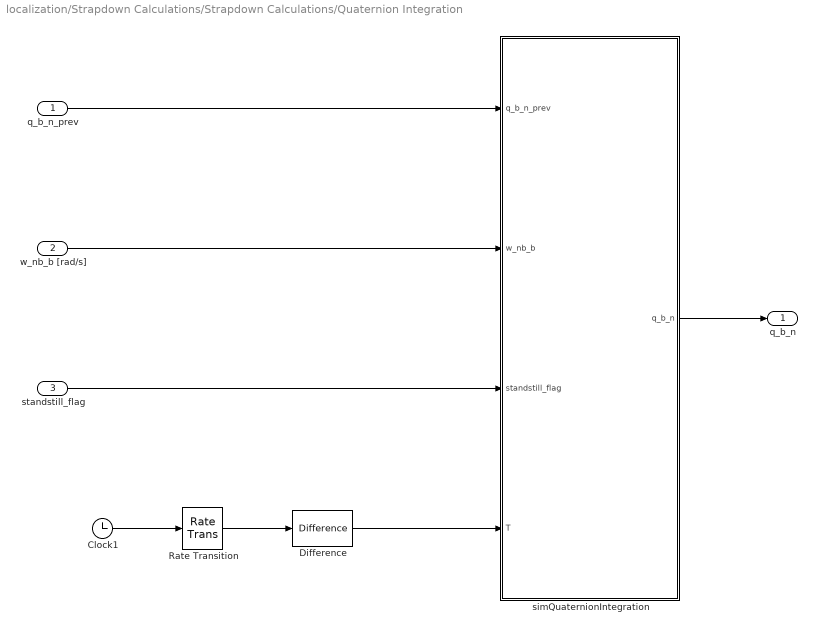
== system localization/Strapdown Calculations/Strapdown Calculations/Quaternion Integration ==
  q_b_n_prev : Inport
  w_nb_b [rad/s] : Inport  Port=2
  standstill_flag : Inport  Port=3
  Clock1 : Clock
  Difference : simulink/Discrete/Difference  ICPrevInput=0.0  OutMin=[]  OutMax=[]  OutDataType=fixdt(1, 16)  OutScaling=2^-10  DoSatur=off
  Rate Transition : RateTransition
  simQuaternionIntegration : MATLAB Function
  q_b_n : Outport  VectorParamsAs1DForOutWhenUnconnected=off
  wires:
  Difference/1 -> simQuaternionIntegration/4(T)
  standstill_flag/1 -> simQuaternionIntegration/3(standstill_flag)
  w_nb_b [rad/s]/1 -> simQuaternionIntegration/2(w_nb_b)
  q_b_n_prev/1 -> simQuaternionIntegration/1(q_b_n_prev)
  simQuaternionIntegration/1(q_b_n) -> q_b_n/1
  Clock1/1 -> Rate Transition/1
  Rate Transition/1 -> Difference/1

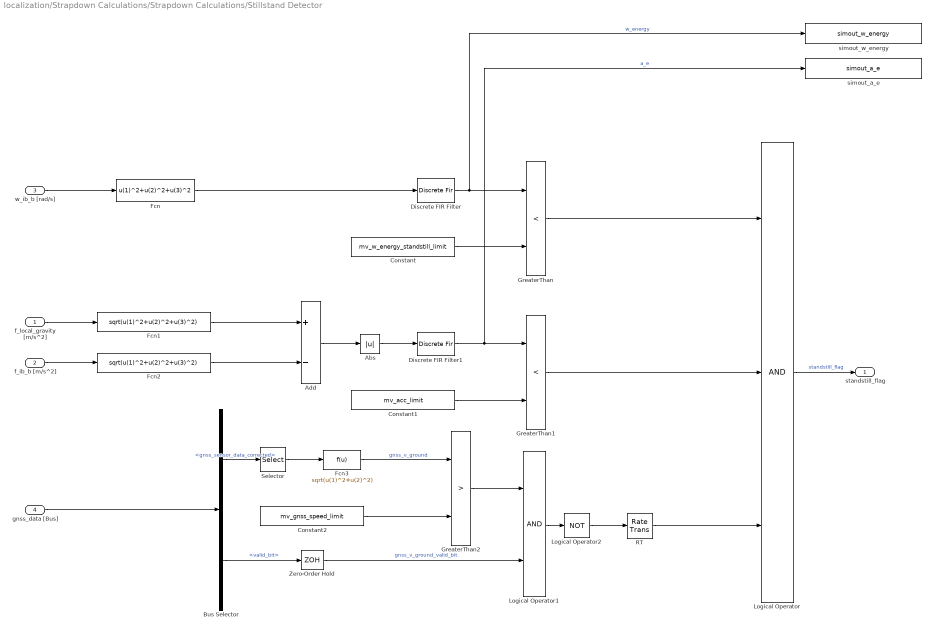
== system localization/Strapdown Calculations/Strapdown Calculations/Stillstand Detector ==
  f_local_gravity [m/s^2] : Inport  SampleTime=sample_time
  f_ib_b [m/s^2] : Inport  Port=2
  w_ib_b [rad/s] : Inport  Port=3
  gnss_data [Bus] : Inport  Port=4
  Abs : Abs
  Add : Sum  Inputs=+-
  Bus Selector : BusSelector  OutputSignals=gnss_sensor_data_corrected,valid_bit
  Constant : Constant  Value=mv_w_energy_standstill_limit
  Constant1 : Constant  Value=mv_acc_limit
  Constant2 : Constant  Value=mv_gnss_speed_limit
  Discrete FIR Filter : DiscreteFir  Coefficients=ones(1,ceil(mv_E_w_ma_time/sample_time))*1/ceil(mv_E_w_ma_time/sample_time)
  Discrete FIR Filter1 : DiscreteFir  Coefficients=ones(1,ceil(mv_a_e_ma_time/sample_time))*1/ceil(mv_a_e_ma_time/sample_time)
  Fcn : Fcn  Expr=u(1)^2+u(2)^2+u(3)^2
  Fcn1 : Fcn  Expr=sqrt(u(1)^2+u(2)^2+u(3)^2)
  Fcn2 : Fcn  Expr=sqrt(u(1)^2+u(2)^2+u(3)^2)
  Fcn3 : Fcn  Expr=sqrt(u(1)^2+u(2)^2)
  GreaterThan : RelationalOperator  Operator=<  OutDataTypeStr=boolean  RndMeth=Simplest
  GreaterThan1 : RelationalOperator  Operator=<  OutDataTypeStr=boolean  RndMeth=Simplest
  GreaterThan2 : RelationalOperator  Operator=>  OutDataTypeStr=boolean  RndMeth=Simplest
  Logical Operator : Logic  Inputs=3  AllPortsSameDT=off  OutDataTypeStr=boolean
  Logical Operator1 : Logic  AllPortsSameDT=off  OutDataTypeStr=boolean
  Logical Operator2 : Logic  Operator=NOT  AllPortsSameDT=off  OutDataTypeStr=boolean
  RT : RateTransition
  Selector : Selector  InputPortWidth=7  IndexOptions=Index vector (dialog)  Indices=[4:6]  OutputSizes=1
  Zero-Order Hold : ZeroOrderHold  SampleTime=gnss_sample_time
  simout_a_e : ToWorkspace  VariableName=simout_a_e  SaveFormat=Timeseries  SampleTime=-1
  simout_w_energy : ToWorkspace  VariableName=simout_w_energy  SaveFormat=Timeseries  SampleTime=-1
  standstill_flag : Outport
  wires:
  Discrete FIR Filter/1 -> simout_w_energy/1, GreaterThan/1  "w_energy"
  Fcn/1 -> Discrete FIR Filter/1
  w_ib_b [rad/s]/1 -> Fcn/1
  Constant/1 -> GreaterThan/2
  GreaterThan/1 -> Logical Operator/1
  Constant1/1 -> GreaterThan1/2
  Discrete FIR Filter1/1 -> simout_a_e/1, GreaterThan1/1  "a_e"
  Logical Operator/1 -> standstill_flag/1  "standstill_flag"
  GreaterThan1/1 -> Logical Operator/2
  Abs/1 -> Discrete FIR Filter1/1
  Fcn1/1 -> Add/1
  Fcn2/1 -> Add/2
  Add/1 -> Abs/1
  f_ib_b [m/s^2]/1 -> Fcn2/1
  f_local_gravity [m/s^2]/1 -> Fcn1/1
  Bus Selector/1 -> Selector/1  "<gnss_sensor_data_corrected>"
  Bus Selector/2 -> Zero-Order Hold/1  "<valid_bit>"
  gnss_data [Bus]/1 -> Bus Selector/1
  Selector/1 -> Fcn3/1
  Fcn3/1 -> GreaterThan2/1  "gnss_v_ground"
  Constant2/1 -> GreaterThan2/2
  GreaterThan2/1 -> Logical Operator1/1
  Zero-Order Hold/1 -> Logical Operator1/2  "gnss_v_ground_valid_bit"
  Logical Operator1/1 -> Logical Operator2/1
  Logical Operator2/1 -> RT/1
  RT/1 -> Logical Operator/3

== system localization/Strapdown Calculations/Strapdown Calculations/Vehicle Position ==
  "p_llh_b_n [rad, rad, m]" : Inport
  Mux : Mux  Inputs=2
  Selector : Selector  InputPortWidth=3  IndexOptions=Index vector (dialog)  Indices=[1 2]  OutputSizes=1
  Selector1 : Selector  InputPortWidth=3  IndexOptions=Index vector (dialog)  Indices=3  OutputSizes=1
  radToDeg : Gain  Gain=180/pi
  "p_llh_b_n [deg, deg, m]" : Outport  VectorParamsAs1DForOutWhenUnconnected=off
  wires:
  "p_llh_b_n [rad, rad, m]"/1 -> Selector1/1, Selector/1
  Selector1/1 -> Mux/2
  Selector/1 -> radToDeg/1
  Mux/1 -> "p_llh_b_n [deg, deg, m]"/1
  radToDeg/1 -> Mux/1

== matlab function localization/Localization Filter/MATLAB Function ==
  data: u input; y output
function y = fcn(u)

x_new = [u(1:3);0;0;u(6);0];

y = repmat(x_new,1,3);

end % function

== matlab function localization/Localization Filter/MATLAB Function2 ==
  data: u input; y output
function y = fcn(u)

coder.extrinsic('simplifyHeadingD');
y = coder.nullcopy(zeros(1,1));

y = deg2rad(simplifyHeadingD(rad2deg(u),'180'));

end % function

== matlab function localization/Localization Filter/Prepare Filter Data ==
  data: u output; gnss_data input; z output; a_eb_n input; w_nb_b input; attitude_deg input; gnss_lever_arm_b input; gnss_uncertainties input; imu_uncertainties input; R output; p_0_utm output; gnss_valid_flag output
function [u,z,R,p_0_utm,gnss_valid_flag] = simFcn_PrepareFilterData(gnss_data,a_eb_n,w_nb_b,attitude_deg,gnss_lever_arm_b,gnss_uncertainties,imu_uncertainties)

x = coder.nullcopy(zeros(1,1));
y = coder.nullcopy(zeros(1,1));
utm_zone = coder.nullcopy(zeros(1,1));

persistent p_0_utm_mem_var

%% Init

if isempty(p_0_utm_mem_var)
    [x,y,utm_zone]=ll2utm_stripped(gnss_data(1),gnss_data(2));
    p_0_utm_mem_var = [x;y;utm_zone];
end % if

imu_data = [a_eb_n;w_nb_b];

%% Calc

% GNSS data _______________________________________________________________

gnss_valid_flag = gnss_data(8);

if gnss_valid_flag
    
    [x,y]=ll2utm_stripped(gnss_data(1),gnss_data(2),p_0_utm_mem_var(3));
    x = x - p_0_utm_mem_var(1);
    y = y - p_0_utm_mem_var(2);
    p_gnss = [x;y];
    % p_gnss_corrected = correctGnssOffset(p_gnss,gnss_lever_arm_b,attitude_deg);
    p_gnss_corrected = p_gnss;
    v_ground = sqrt(sum(gnss_data([4,5]).^2));
    psi = deg2rad(gnss_data(7));
    
    z_gnss = [p_gnss_corrected;v_ground;psi];    
    R_gnss = diag(gnss_uncertainties([2,1,3,4]).^2);
    
else
    
    z_gnss = zeros(4,1);
    R_gnss = zeros(4,4);
    
end % if

% IMU data ________________________________________________________________

% Extract direction
psi_acc = atan2d(imu_data(2),imu_data(1));
psi_strapdown = attitude_deg(3);
if abs(angdiff(deg2rad(psi_acc),deg2rad(psi_strapdown))) <= pi/2
    dir = 1;
else
    dir = -1;
end % if

% IMU data
a_ground = dir * sqrt(sum(imu_data([1,2]).^2));
w = imu_data(6);

% Collection
z_imu = [a_ground;w];
R_imu = diag([imu_uncertainties(1), imu_uncertainties(2)].^2);

%% Output

u = 0;
z = [z_gnss;z_imu];
R = blkdiag(R_gnss,R_imu);

p_0_utm = p_0_utm_mem_var;

end % function

%% Helper Functions

function p_gnss_corrected = correctGnssOffset(p_gnss,gnss_lever_arm_b,attitude_deg)

q_b_n = eulerToQuat(deg2rad(attitude_deg));
gnss_lever_arm_n = transformVect(gnss_lever_arm_b,q_b_n);

p_gnss_corrected = p_gnss(:)-[0 1;1 0]*gnss_lever_arm_n(1:2);

% yaw_rad = deg2rad(attitude_deg(3));
% rot_matrix = @(psi) [cos(psi-pi/2) sin(psi-pi/2);-sin(psi-pi/2) cos(psi-pi/2)];
% 
% p_gnss_corrected = p_gnss(:)-rot_matrix(yaw_rad)*gnss_lever_arm_b(1:2);

end % if

== matlab function localization/Localization Filter/MATLAB Function1 ==
  data: u input; y output
function y = fcn(u)

y = cat(3,u,u,u);

end % function

== matlab function localization/Localization Filter/Parameter Identification, Localization Correction and Map Building/Correction/MATLAB Function ==
  data: enable input; reset_flag input; x_imm input; s output; P_x_imm input; s_0 input; P_s_0 input; z_s input; R_s input; Q_straight input; Q_arc input; geometry input; P_s output; o output; P_o output
function [s,P_s,o,P_o] = simFcn_Correction(enable,reset_flag,x_imm,P_x_imm,s_0,P_s_0,z_s,R_s,Q_straight,Q_arc,geometry)

% Init ____________________________________________________________________

s = coder.nullcopy(zeros(8,1));
P_s = coder.nullcopy(zeros(8,8));
o = coder.nullcopy(zeros(4,1));
P_o = coder.nullcopy(zeros(4,4));

% Calculations ____________________________________________________________

[s,P_s,o,P_o] = simFcn_TgcCorrection(enable,reset_flag,x_imm,P_x_imm,s_0,P_s_0,z_s,R_s,Q_straight,Q_arc,geometry);

end % function
